simulink model "Centrifugal_Pump"  (R2023a)
settings: Solver=VariableStepAuto  StartTime=0.0  StopTime=simtime  MaxStep=0.01  RelTol=1e-4
values from neighbouring files (symbols this model uses):
  J_CFP = 0.02    [Model_Values.mat]
  J_Fl = 0.7    [Model_Values.mat]
  k = 6    [Model_Values.mat]
  k_CFP = 10    [Model_Values.mat]
  M_in = 0.003    [Model_Values.mat]
  R_CFP = 6    [Model_Values.mat]
settings Model: Creator=fycce  LastModifiedBy=fycce
settings DataIOCC: SaveOutput=off  SaveTime=off  ReturnWorkspaceOutputs=off

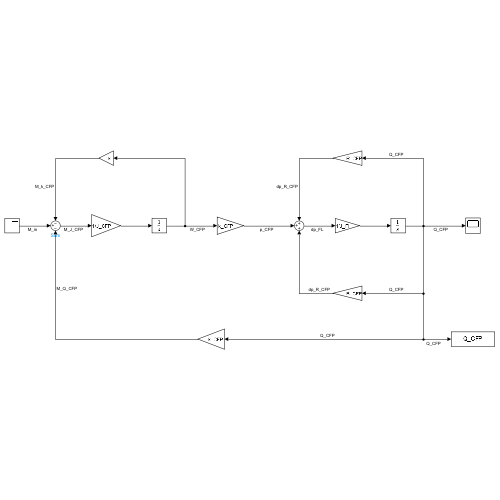
[thumbnail: Simulink's stored preview of the top-level diagram]
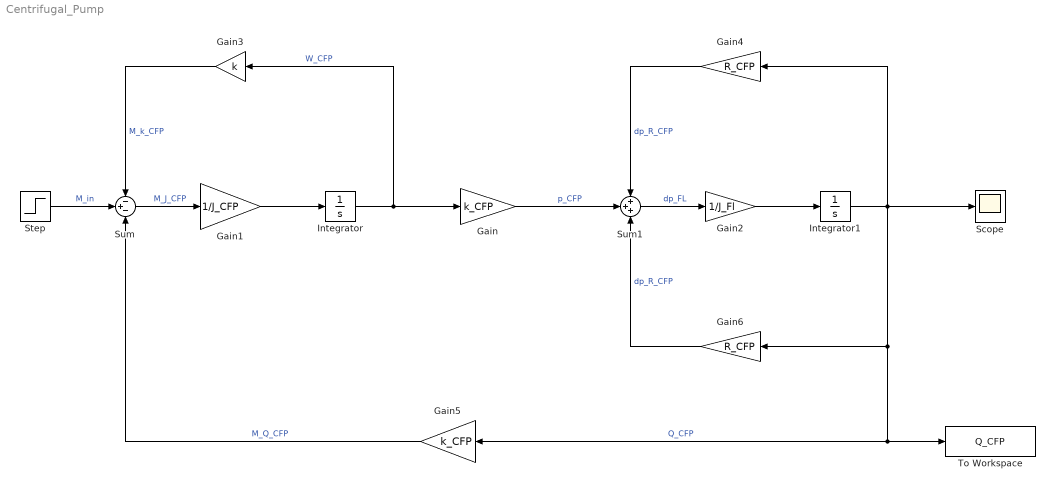
== system Centrifugal_Pump ==
  Gain : Gain  Gain=k_CFP
  Gain1 : Gain  Gain=1/J_CFP
  Gain2 : Gain  Gain=1/J_Fl
  Gain3 : Gain  Gain=k
  Gain4 : Gain  Gain=R_CFP
  Gain5 : Gain  Gain=k_CFP
  Gain6 : Gain  Gain=R_CFP
  Integrator : Integrator
  Integrator1 : Integrator
  Scope : Scope
  Step : Step  After=M_in  SampleTime=0
  Sum : Sum  Inputs=-+-
  Sum1 : Sum  Inputs=+++
  To Workspace : ToWorkspace  VariableName=Q_CFP  SaveFormat=Timeseries  SampleTime=-1
  wires:
  Step/1 -> Sum/2  "M_in"
  Gain/1 -> Sum1/2  "p_CFP"
  Integrator/1 -> Gain3/1, Gain/1  "W_CFP"
  Sum/1 -> Gain1/1  "M_J_CFP"
  Gain1/1 -> Integrator/1
  Gain2/1 -> Integrator1/1
  Sum1/1 -> Gain2/1  "dp_FL"
  Integrator1/1 -> Gain4/1, Scope/1, To Workspace/1, Gain5/1, Gain6/1  "Q_CFP"
  Gain3/1 -> Sum/1  "M_k_CFP"
  Gain4/1 -> Sum1/1  "dp_R_CFP"
  Gain5/1 -> Sum/3  "M_Q_CFP"
  Gain6/1 -> Sum1/3  "dp_R_CFP"
